simulink model "testHierCtrl"  (R2020a)
settings: Solver=FixedStepAuto  StartTime=0.0  StopTime=inf  FixedStep=0.01  RelTol=1e-3  EnableMultiTasking=on
values from neighbouring files (symbols this model uses):
  FLIGHTCONTROLLER = 'periodicCtrlExp'    [openWaterInit.m]
undefined symbols (not defined in the file or in its folder): env, fltCtrl, hiLvlCtrl, initializeBussesFromBlock, vhcl
libraries: simulink x6, filteredPIDController_ul x2, velocityAngle_ul x2, eeGeneralControl x1, stopwatch_ul x1, courseFollowManta_cl x1, ctrlAllocMatrix_cl x1, eulAng2RotMat_ul x1, angleBtw2Vecs_ul x1, vrlib x1, alphaBeta_ul x1, gnd2TanRotation_ul x1
settings Model: SimulationMode=external  Creator=andre  LastModifiedBy=mae-vermillionlab
settings SolverCC: ConcurrentTasks=on  AutoInsertRateTranBlk=on
settings DataIOCC: SaveFormat=StructureWithTime
settings OptimizationCC: BlockReduction=off  OptimizeBlockIOStorage=off
settings HardwareCC: ProdBitPerPointer=32  ProdBitPerSizeT=32  ProdBitPerPtrDiffT=32  ProdLargestAtomicFloat=None  ProdWordSize=32  ProdLongLongMode=on  ProdHWDeviceType=Generic->32-bit x86 compatible
settings RTWCC: Description=Simulink Real-Time  SystemTargetFile=slrt.tlc  TemplateMakefile=slrt_default_tmf  CodeExecutionProfiling=on  RTWCompilerOptimization=on
settings SimulinkRealTimeCC: SupportVariableSizeSignals=on  RL32LogTETModifier=off  xPCConcurrentTasks=on

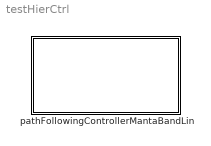
== system testHierCtrl ==
  pathFollowingControllerMantaBandLin : Subsystem  LoadFcn=initializeBussesFromBlock(gcb)  InitFcn=initializeBussesFromBlock(gcb)  StartFcn=initializeBussesFromBlock(gcb)  VariantControl=strcmpi(FLIGHTCONTROLLER,'pathFollowingControllerMantaBandLin')  mask{initPosForInitSStar=vhcl.initPosVecGnd.Value, fluidDensity=env.water.density.Value, pathCtrl=fltCtrl, aeroStruct=vhcl.struct('OCT.aeroSurf')}
      mask prompts: initPosForInitSStar "Initial Position"; fluidDensity "Fluid Density"; pathCtrl "Controller"; aeroStruct "Aerodynamic Structure"
      settings: MinAlgLoopOccurrences=on
      mask DialogControl Container3 Prompt: courseFollow Params
      mask DialogControl Container4 Prompt: setpointToOutput Params

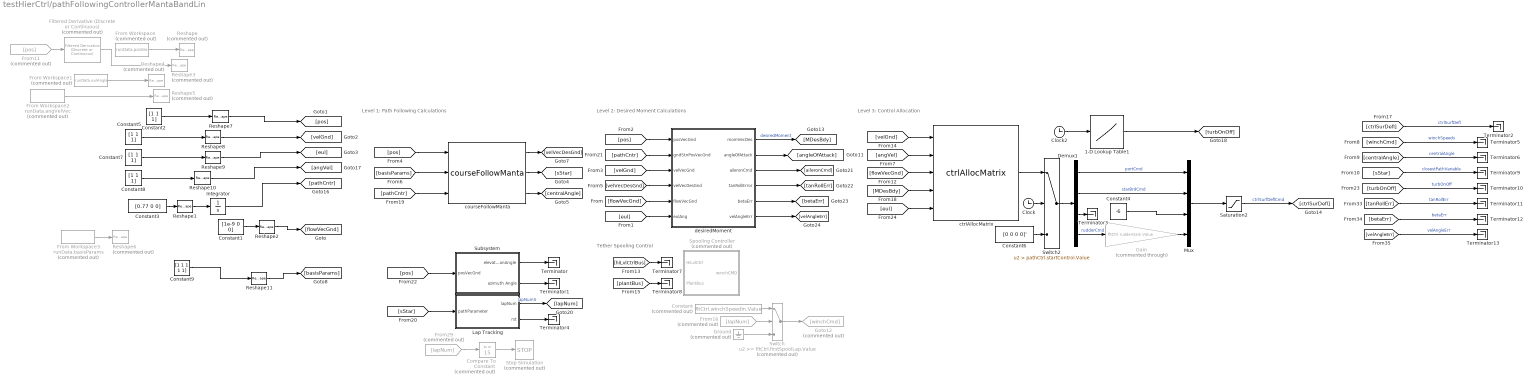
== system testHierCtrl/pathFollowingControllerMantaBandLin ==
  note: Level 1: Path Following Calculations
  note: Level 2: Desired Moment Calculations
  note: Tether Spooling Control
  note: Level 3: Control Allocation
  1-D Lookup Table1 : Lookup_n-D  NumberOfTableDimensions=1  BreakpointsForDimension1=[0 1000 2000]  Table=[0 0 0]  InterpMethod=Flat  InternalRulePriority=Speed  RndMeth=Simplest  InputSameDT=on
  Clock : Clock
  Clock2 : Clock
  Compare To Constant : simulink/Logic and Bit Operations/Compare To Constant  Commented=on  relop=>=  const=15  OutDataTypeStr=boolean
  Constant : Constant  Commented=on  Value=fltCtrl.winchSpeedIn.Value
  Constant1 : Constant  Value=[1e-9 0 0]
  Constant{2,5,7..8} (4 alike) : Constant  Value=[1 1 1]
  Constant3 : Constant  Value=[0.77 0 0]
  Constant4 : Constant  Value=-6
  Constant6 : Constant  Value=[0 0 0 0]'
  Constant9 : Constant  Value=[1 1 1 1 1]
  Demux1 : Demux
  Filtered Derivative (Discrete or Continuous) : eeGeneralControl/Filtered Derivative (Discrete or Continuous)  Commented=on  K=1  T=0.1  B=inf  A=-inf  minRatio=10  init_option=Inherited from block input  x0=0  Ts=-1
      settings: SourceProductBaseCode=PS
  From Workspace : FromWorkspace  Commented=on  VariableName=runData.posVec
  From Workspace1 : FromWorkspace  Commented=on  VariableName=runData.eulAngle
  From Workspace2 : FromWorkspace  Commented=on  VariableName=runData.angVelVec
  From Workspace3 : FromWorkspace  Commented=on  VariableName=runData.basisParams
  From11 : From  Commented=on  GotoTag=pos
  From16 : From  Commented=on  GotoTag=lapNum
  From29 : From  Commented=on  GotoTag=lapNum
  Gain : Gain  Commented=through  Gain=fltCtrl.rudderGain.Value
  Goto12 : Goto  Commented=on  GotoTag=winchCmd
  Ground : Ground  Commented=on
  Integrator : Integrator  InitialCondition=[0 0 0]'
  Lap Tracking : Subsystem
  Mux : Mux
  Reshape{,3..6} (5 alike) : Reshape  Commented=on  OutputDimensionality=Column vector (2-D)
  Reshape{1..2,7..11} (7 alike) : Reshape  OutputDimensionality=Column vector (2-D)
  Saturation2 : Saturate  UpperLimit=pathCtrl.controlSigMax.upperLimit.Value  LowerLimit=pathCtrl.controlSigMax.lowerLimit.Value
  "Spooling Controller " : Subsystem  Commented=on
  Stop Simulation : Stop  Commented=on
  Subsystem : Subsystem
  Switch : Switch  Commented=on  Threshold=fltCtrl.firstSpoolLap.Value
  Switch2 : Switch  Criteria=u2 > Threshold  Threshold=pathCtrl.startControl.Value
  Terminator{,1..13} (14 alike) : Terminator
  courseFollowManta : courseFollowManta_cl/courseFollowManta  SystemSampleTime=-1  Latency=0  AutoFrameSizeCalculation=off
      link override Memory1: InitialCondition=0
  ctrlAllocMatrix : ctrlAllocMatrix_cl/ctrlAllocMatrix  aeroStruct=aeroStruct  fluidDensity=fluidDensity
  desiredMoment : Subsystem
  wires:
  [velAngleErr] -> Terminator13/1  "velAngleErr"
  desiredMoment/6(velAngleErr) -> [velAngleErr]
  [betaErr] -> Terminator12/1  "betaErr"
  [tanRollErr] -> Terminator11/1  "tanRollErr"
  desiredMoment/5(betaErr) -> [betaErr]
  desiredMoment/4(tanRollError) -> [tanRollErr]
  Mux/1 -> Saturation2/1
  desiredMoment/3(aileronCmd) -> [aileronCmd]
  Compare To Constant/1 -> Stop Simulation/1
  From29/1 -> Compare To Constant/1
  Ground/1 -> Switch/3
  Constant/1 -> Switch/1
  From16/1 -> Switch/2
  Switch/1 -> Goto12/1
  [plantBus] -> Terminator8/1
  [hiLvlCtrlBus] -> Terminator7/1
  Lap Tracking/1(lapNum) -> [lapNum]  "lapNumS"
  Lap Tracking/2(rst) -> Terminator4/1
  [sStar] -> Lap Tracking/1(pathParameter)
  Clock2/1 -> 1-D Lookup Table1/1
  1-D Lookup Table1/1 -> [turbOnOff]
  desiredMoment/2(angleOfAttack) -> [angleOfAttack]
  Constant4/1 -> Mux/3
  Subsystem/2(azimuth Angle) -> Terminator1/1
  Subsystem/1(elevationAngle) -> Terminator/1
  [pos] -> Subsystem/1(posVecGnd)
  [turbOnOff] -> Terminator10/1  "turbOnOff"
  Demux1/4 -> Gain/1  "rudderCmd"
  Gain/1 -> Mux/4
  [basisParams] -> courseFollowManta/2
  [flowVecGnd] -> desiredMoment/5(flowVecGnd)
  [eul] -> desiredMoment/6(eulAng)
  [velVecDesGnd] -> desiredMoment/4(velVecDesGnd)
  [velGnd] -> desiredMoment/3(velVecGnd)
  [pathCntr] -> desiredMoment/2(gndStnPosVecGnd)
  [pos] -> desiredMoment/1(posVecGnd)
  [pathCntr] -> courseFollowManta/3
  [eul] -> ctrlAllocMatrix/5
  Saturation2/1 -> [ctrlSurDefl]  "ctrlSurfDeflCmd"
  [ctrlSurDefl] -> Terminator2/1  "ctrlSurfDefl"
  ctrlAllocMatrix/1 -> Switch2/1
  [MDesBdy] -> ctrlAllocMatrix/4
  Constant6/1 -> Switch2/3
  Switch2/1 -> Demux1/1
  Clock/1 -> Switch2/2
  Demux1/2 -> Mux/2  "starBrdCmd"
  Demux1/1 -> Mux/1  "portCmd"
  Demux1/3 -> Terminator3/1
  [flowVecGnd] -> ctrlAllocMatrix/3
  [velGnd] -> ctrlAllocMatrix/1
  [angVel] -> ctrlAllocMatrix/2
  desiredMoment/1(momVecDes) -> [MDesBdy]  "desiredMoment"
  courseFollowManta/3 -> [centralAngle]
  [sStar] -> Terminator9/1  "closestPathVariable"
  [centralAngle] -> Terminator6/1  "centralAngle"
  courseFollowManta/2 -> [sStar]
  [winchCmd] -> Terminator5/1  "winchSpeeds"
  [pos] -> courseFollowManta/1
  courseFollowManta/1 -> [velVecDesGnd]
  From Workspace/1 -> Reshape/1
  Filtered Derivative (Discrete or Continuous)/1 -> Reshape3/1
  From Workspace1/1 -> Reshape4/1
  Constant3/1 -> Reshape1/1
  Reshape1/1 -> Integrator/1
  Constant1/1 -> Reshape2/1
  Reshape2/1 -> [flowVecGnd]
  From11/1 -> Filtered Derivative (Discrete or Continuous)/1
  From Workspace2/1 -> Reshape5/1
  From Workspace3/1 -> Reshape6/1
  Reshape7/1 -> [pos]
  Constant2/1 -> Reshape7/1
  Constant5/1 -> Reshape8/1
  Constant7/1 -> Reshape9/1
  Constant8/1 -> Reshape10/1
  Integrator/1 -> [pathCntr]
  Reshape10/1 -> [angVel]
  Reshape9/1 -> [eul]
  Reshape8/1 -> [velGnd]
  Reshape11/1 -> [basisParams]
  Constant9/1 -> Reshape11/1

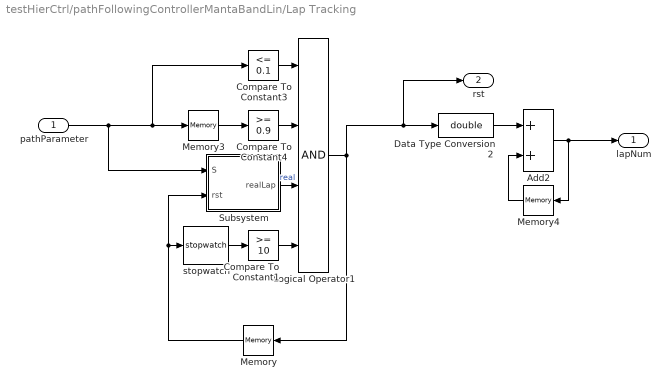
== system testHierCtrl/pathFollowingControllerMantaBandLin/Lap Tracking ==
  pathParameter : Inport
  Add2 : Sum
  Compare To Constant1 : simulink/Logic and Bit Operations/Compare To Constant  relop=>=  const=10  OutDataTypeStr=boolean
  Compare To Constant3 : simulink/Logic and Bit Operations/Compare To Constant  relop=<=  const=0.1  OutDataTypeStr=boolean
  Compare To Constant4 : simulink/Logic and Bit Operations/Compare To Constant  relop=>=  const=0.9  OutDataTypeStr=boolean
  Data Type Conversion2 : DataTypeConversion  OutDataTypeStr=double
  Logical Operator1 : Logic  Inputs=4  AllPortsSameDT=off  OutDataTypeStr=boolean
  Memory : Memory  InitialCondition=false
  Memory3 : Memory
  Memory4 : Memory
  Subsystem : Subsystem
  stopwatch : stopwatch_ul/stopwatch  SystemSampleTime=-1  Latency=0  AutoFrameSizeCalculation=off
  lapNum : Outport  VectorParamsAs1DForOutWhenUnconnected=off
  rst : Outport  Port=2  VectorParamsAs1DForOutWhenUnconnected=off
  wires:
  Subsystem/1(realLap) -> Logical Operator1/3  "real"
  Compare To Constant1/1 -> Logical Operator1/4
  Memory/1 -> stopwatch/1, Subsystem/2(rst)
  stopwatch/1 -> Compare To Constant1/1
  pathParameter/1 -> Memory3/1, Compare To Constant3/1, Subsystem/1(S)
  Compare To Constant4/1 -> Logical Operator1/2
  Add2/1 -> Memory4/1, lapNum/1
  Memory4/1 -> Add2/2
  Logical Operator1/1 -> Memory/1, Data Type Conversion2/1, rst/1
  Data Type Conversion2/1 -> Add2/1
  Memory3/1 -> Compare To Constant4/1
  Compare To Constant3/1 -> Logical Operator1/1

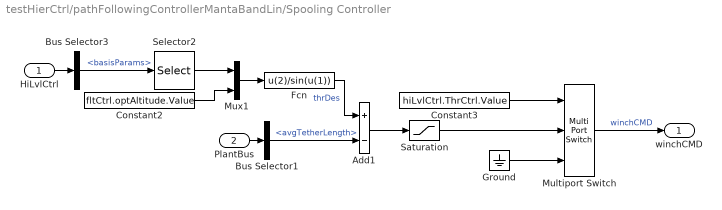
== system testHierCtrl/pathFollowingControllerMantaBandLin/Spooling Controller  ==
  HiLvlCtrl : Inport
  PlantBus : Inport  Port=2
  Add1 : Sum  Inputs=+-
  Bus Selector1 : BusSelector  OutputSignals=avgTetherLength
  Bus Selector3 : BusSelector  OutputSignals=basisParams
  Constant2 : Constant  Value=fltCtrl.optAltitude.Value
  Constant3 : Constant  Value=hiLvlCtrl.ThrCtrl.Value
  Fcn : Fcn  Expr=u(2)/sin(u(1))
  Ground : Ground
  Multiport Switch : MultiPortSwitch  DataPortOrder=Specify indices  Inputs=2  DataPortIndices={0,1}
  Mux1 : Mux  Inputs=2
  Saturation : Saturate  UpperLimit=.25  LowerLimit=-.25
  Selector2 : Selector  InputPortWidth=5  IndexOptions=Index vector (dialog)  Indices=3  OutputSizes=1
  winchCMD : Outport
  wires:
  PlantBus/1 -> Bus Selector1/1
  Constant3/1 -> Multiport Switch/1
  Saturation/1 -> Multiport Switch/2
  Ground/1 -> Multiport Switch/3
  HiLvlCtrl/1 -> Bus Selector3/1
  Multiport Switch/1 -> winchCMD/1  "winchCMD"
  Selector2/1 -> Mux1/1
  Fcn/1 -> Add1/1  "thrDes"
  Add1/1 -> Saturation/1
  Constant2/1 -> Mux1/2
  Bus Selector1/1 -> Add1/2  "<avgTetherLength>"
  Mux1/1 -> Fcn/1
  Bus Selector3/1 -> Selector2/1  "<basisParams>"

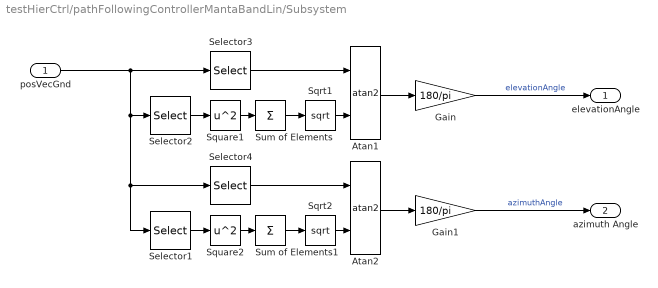
== system testHierCtrl/pathFollowingControllerMantaBandLin/Subsystem ==
  posVecGnd : Inport
  Atan1 : Trigonometry  Operator=atan2
  Atan2 : Trigonometry  Operator=atan2
  Gain : Gain  Gain=180/pi
  Gain1 : Gain  Gain=180/pi
  Selector1 : Selector  InputPortWidth=3  IndexOptions=Index vector (dialog)  Indices=1  OutputSizes=1
  Selector2 : Selector  InputPortWidth=3  IndexOptions=Index vector (dialog)  Indices=[1 2]  OutputSizes=1
  Selector3 : Selector  InputPortWidth=3  IndexOptions=Index vector (dialog)  Indices=3  OutputSizes=1
  Selector4 : Selector  InputPortWidth=3  IndexOptions=Index vector (dialog)  Indices=2  OutputSizes=1
  Sqrt1 : Sqrt  SaturateOnIntegerOverflow=on
  Sqrt2 : Sqrt  SaturateOnIntegerOverflow=on
  Square1 : Math  Operator=square  SignedPower=on  SaturateOnIntegerOverflow=on
  Square2 : Math  Operator=square  SignedPower=on  SaturateOnIntegerOverflow=on
  Sum of Elements : Sum  Inputs=+
  Sum of Elements1 : Sum  Inputs=+
  elevationAngle : Outport
  azimuth Angle : Outport  Port=2
  wires:
  Gain1/1 -> azimuth Angle/1  "azimuthAngle"
  Selector4/1 -> Atan2/1
  Sqrt2/1 -> Atan2/2
  posVecGnd/1 -> Selector3/1, Selector2/1, Selector4/1, Selector1/1
  Selector1/1 -> Square2/1
  Sum of Elements1/1 -> Sqrt2/1
  Square2/1 -> Sum of Elements1/1
  Atan2/1 -> Gain1/1
  Gain/1 -> elevationAngle/1  "elevationAngle"
  Selector2/1 -> Square1/1
  Atan1/1 -> Gain/1
  Sum of Elements/1 -> Sqrt1/1
  Selector3/1 -> Atan1/1
  Square1/1 -> Sum of Elements/1
  Sqrt1/1 -> Atan1/2

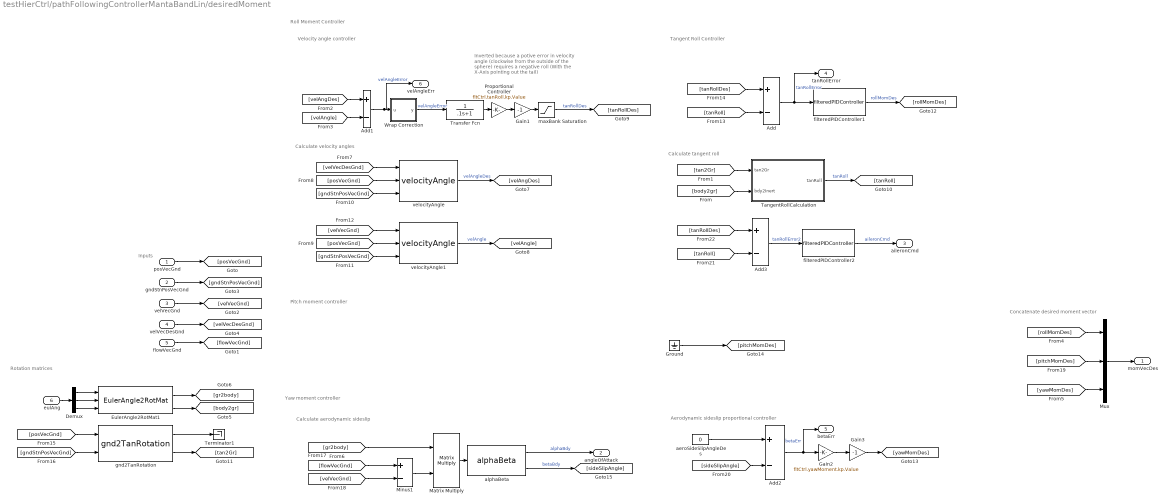
== system testHierCtrl/pathFollowingControllerMantaBandLin/desiredMoment ==
  note: Calculate aerodynamic sideslip
  note: Aerodynamic sideslip proportional controller
  note: Roll Moment Controller
  note: Concatenate desired moment vector
  note: Tangent Roll Controller
  note: Calculate tangent roll
  note: Calculate velocity angles
  note: Rotation matrices
  note: Inputs
  note: Velocity angle controller
  note: Inverted because a potive error
      | in velocity angle (clockwise from the
      | outside of the sphere) requires a negative
      | roll (With the X-Axis pointing out the tail)
  note: Pitch moment controller
  note: Yaw moment controller
  posVecGnd : Inport
  gndStnPosVecGnd : Inport  Port=2
  velVecGnd : Inport  Port=3
  velVecDesGnd : Inport  Port=4
  flowVecGnd : Inport  Port=5
  eulAng : Inport  Port=6
  Add{,1..3} (4 alike) : Sum  Inputs=+-
  Demux : Demux  Outputs=3
  EulerAngle2RotMat1 : eulAng2RotMat_ul/EulerAngle2RotMat  SystemSampleTime=-1  Latency=0  AutoFrameSizeCalculation=off
  Gain1 : Gain  Gain=-1
  Gain2 : Gain  Gain=fltCtrl.yawMoment.kp.Value
  Gain3 : Gain  Gain=-1
  Ground : Ground
  Matrix Multiply : Product  Multiplication=Matrix(*)
  Minus1 : Sum  Inputs=+-
  Mux : Mux  Inputs=3
  Proportional Controller : Gain  Gain=fltCtrl.tanRoll.kp.Value
  TangentRollCalculation : Subsystem
  Terminator1 : Terminator
  Transfer Fcn : TransferFcn  Denominator=[.1 1]
  Wrap Correction : Subsystem
  aeroSideSlipAngleDes : Constant  Value=0
  alphaBeta : alphaBeta_ul/alphaBeta  SystemSampleTime=-1  Latency=0  AutoFrameSizeCalculation=off
  filteredPIDController1 : filteredPIDController_ul/filteredPIDController  kp=pathCtrl.rollMoment.kp.Value  ki=0  kd=pathCtrl.rollMoment.kd.Value  Value=pathCtrl.rollMoment.tau.Value  externalReset=none
  filteredPIDController2 : filteredPIDController_ul/filteredPIDController  kp=fltCtrl.rollCtrl.kp.Value  ki=fltCtrl.rollCtrl.ki.Value  kd=fltCtrl.rollCtrl.kd.Value  Value=fltCtrl.rollCtrl.tau.Value  externalReset=none
  gnd2TanRotation : gnd2TanRotation_ul/gnd2TanRotation  SystemSampleTime=-1  Latency=0  AutoFrameSizeCalculation=off
  maxBank Saturation : Saturate  UpperLimit=pathCtrl.maxBank.upperLimit.Value  LowerLimit=pathCtrl.maxBank.lowerLimit.Value
  velocityAngle : velocityAngle_ul/velocityAngle  SystemSampleTime=-1  Latency=0  AutoFrameSizeCalculation=off
  velocityAngle1 : velocityAngle_ul/velocityAngle  SystemSampleTime=-1  Latency=0  AutoFrameSizeCalculation=off
  momVecDes : Outport  VectorParamsAs1DForOutWhenUnconnected=off
  angleOfAttack : Outport  Port=2  VectorParamsAs1DForOutWhenUnconnected=off
  aileronCmd : Outport  Port=3  VectorParamsAs1DForOutWhenUnconnected=off
  tanRollError : Outport  Port=4
  betaErr : Outport  Port=5
  velAngleErr : Outport  Port=6
  wires:
  filteredPIDController2/1 -> aileronCmd/1  "aileronCmd"
  [tanRollDes] -> Add3/1
  [tanRoll] -> Add3/2
  Add3/1 -> filteredPIDController2/1  "tanRollError2"
  Transfer Fcn/1 -> Proportional Controller/1
  Wrap Correction/1(y) -> Transfer Fcn/1  "velAngleError"
  Ground/1 -> [pitchMomDes]
  posVecGnd/1 -> [posVecGnd]
  velVecGnd/1 -> [velVecGnd]
  Add/1 -> filteredPIDController1/1, tanRollError/1  "tanRollError"
  Proportional Controller/1 -> Gain1/1
  Gain1/1 -> maxBank Saturation/1
  maxBank Saturation/1 -> [tanRollDes]  "tanRollDes"
  Add1/1 -> velAngleErr/1, Wrap Correction/1(u)  "velAngleError"
  flowVecGnd/1 -> [flowVecGnd]
  [tan2Gr] -> TangentRollCalculation/1(tan2Gr)
  TangentRollCalculation/1(tanRoll) -> [tanRoll]  "tanRoll"
  filteredPIDController1/1 -> [rollMomDes]  "rollMomDes"
  Gain2/1 -> Gain3/1
  Minus1/1 -> Matrix Multiply/2
  [velVecGnd] -> Minus1/2
  [flowVecGnd] -> Minus1/1
  eulAng/1 -> Demux/1
  Demux/3 -> EulerAngle2RotMat1/3
  Demux/1 -> EulerAngle2RotMat1/1
  Demux/2 -> EulerAngle2RotMat1/2
  EulerAngle2RotMat1/2 -> [body2gr]
  EulerAngle2RotMat1/1 -> [gr2body]
  [body2gr] -> TangentRollCalculation/2(bdy2Inert)
  [gr2body] -> Matrix Multiply/1
  Matrix Multiply/1 -> alphaBeta/1
  alphaBeta/2 -> [sideSlipAngle]  "betaBdy"
  Add2/1 -> Gain2/1, betaErr/1  "betaErr"
  aeroSideSlipAngleDes/1 -> Add2/1
  Mux/1 -> momVecDes/1
  Gain3/1 -> [yawMomDes]
  alphaBeta/1 -> angleOfAttack/1  "alphaBdy"
  [pitchMomDes] -> Mux/2
  gndStnPosVecGnd/1 -> [gndStnPosVecGnd]
  velVecDesGnd/1 -> [velVecDesGnd]
  velocityAngle/1 -> [velAngDes]  "velAngleDes"
  velocityAngle1/1 -> [velAngle]  "velAngle"
  [velAngDes] -> Add1/1
  [velAngle] -> Add1/2
  [velVecDesGnd] -> velocityAngle/1
  [posVecGnd] -> velocityAngle/2
  [posVecGnd] -> velocityAngle1/2
  [gndStnPosVecGnd] -> velocityAngle/3
  [gndStnPosVecGnd] -> velocityAngle1/3
  [velVecGnd] -> velocityAngle1/1
  [tanRoll] -> Add/2
  [tanRollDes] -> Add/1
  [posVecGnd] -> gnd2TanRotation/1
  [gndStnPosVecGnd] -> gnd2TanRotation/2
  gnd2TanRotation/2 -> [tan2Gr]
  gnd2TanRotation/1 -> Terminator1/1
  [rollMomDes] -> Mux/1
  [yawMomDes] -> Mux/3
  [sideSlipAngle] -> Add2/2

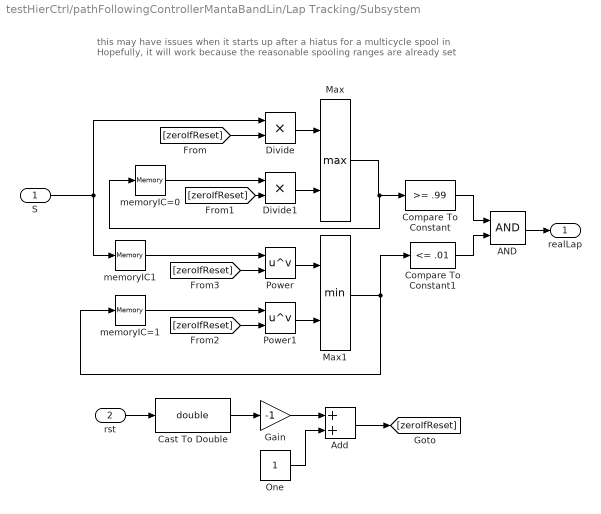
== system testHierCtrl/pathFollowingControllerMantaBandLin/Lap Tracking/Subsystem ==
  note: this may have issues when it starts up after a hiatus for a multicycle spool in
      | Hopefully, it will work because the reasonable spooling ranges are already set
  S : Inport
  rst : Inport  Port=2
  AND : Logic  AllPortsSameDT=off  OutDataTypeStr=boolean
  Add : Sum
  Cast To Double : DataTypeConversion  OutDataTypeStr=double
  Compare To Constant : simulink/Logic and Bit Operations/Compare To Constant  relop=>=  const=.99  OutDataTypeStr=boolean
  Compare To Constant1 : simulink/Logic and Bit Operations/Compare To Constant  relop=<=  const=.01  OutDataTypeStr=boolean
  Divide : Product  Inputs=**
  Divide1 : Product  Inputs=**
  Gain : Gain  Gain=-1
  Max : MinMax  Function=max  Inputs=2
  Max1 : MinMax  Inputs=2
  One : Constant  OutDataTypeStr=Inherit: Inherit via back propagation
  Power : Math  Operator=pow  SaturateOnIntegerOverflow=on
  Power1 : Math  Operator=pow  SaturateOnIntegerOverflow=on
  memoryIC1 : Memory  InitialCondition=1
  memoryIC=0 : Memory
  memoryIC=1 : Memory  InitialCondition=1
  realLap : Outport
  wires:
  memoryIC1/1 -> Power/1
  memoryIC=1/1 -> Power1/1
  [zeroIfReset] -> Power1/2
  memoryIC=0/1 -> Divide1/1
  Divide1/1 -> Max/2
  [zeroIfReset] -> Divide1/2
  [zeroIfReset] -> Power/2
  [zeroIfReset] -> Divide/2
  AND/1 -> realLap/1
  Compare To Constant1/1 -> AND/2
  Compare To Constant/1 -> AND/1
  Cast To Double/1 -> Gain/1
  Power1/1 -> Max1/2
  Power/1 -> Max1/1
  Max/1 -> Compare To Constant/1, memoryIC=0/1
  Divide/1 -> Max/1
  One/1 -> Add/2
  Add/1 -> [zeroIfReset]
  Gain/1 -> Add/1
  S/1 -> memoryIC1/1, Divide/1
  rst/1 -> Cast To Double/1
  Max1/1 -> memoryIC=1/1, Compare To Constant1/1

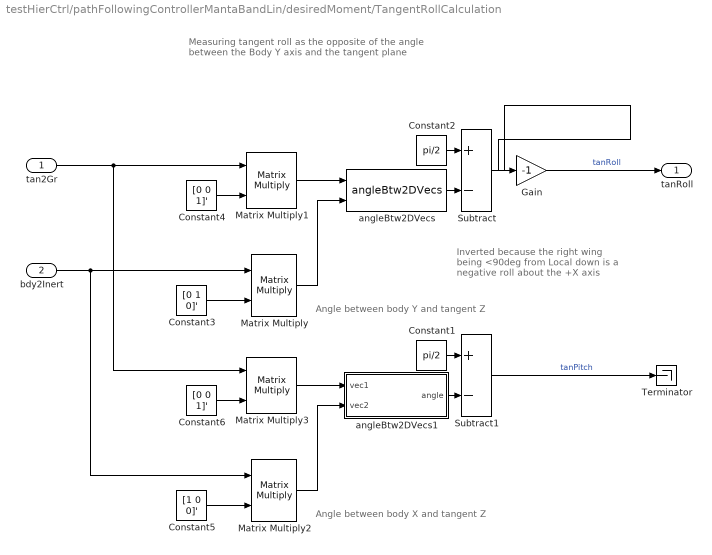
== system testHierCtrl/pathFollowingControllerMantaBandLin/desiredMoment/TangentRollCalculation ==
  note: Measuring tangent roll as the opposite
      | of the angle between the Body Y axis
      | and the tangent plane
  note: Angle between body Y and tangent Z
  note: Inverted because the right wing
      | being <90deg from Local down
      | is a negative roll about the +X axis
  note: Angle between body X and tangent Z
  tan2Gr : Inport
  bdy2Inert : Inport  Port=2
  Constant1 : Constant  Value=pi/2
  Constant2 : Constant  Value=pi/2
  Constant3 : Constant  Value=[0 1 0]'
  Constant4 : Constant  Value=[0 0 1]'
  Constant5 : Constant  Value=[1 0 0]'
  Constant6 : Constant  Value=[0 0 1]'
  Gain : Gain  Gain=-1
  Matrix Multiply{,1..3} (4 alike) : Product  Multiplication=Matrix(*)
  Subtract : Sum  Inputs=+-
  Subtract1 : Sum  Inputs=+-
  Terminator : Terminator
  angleBtw2DVecs : angleBtw2Vecs_ul/angleBtw2DVecs  SystemSampleTime=-1  Latency=0  AutoFrameSizeCalculation=off
  angleBtw2DVecs1 : Subsystem
  tanRoll : Outport  VectorParamsAs1DForOutWhenUnconnected=off
  wires:
  Subtract/1 -> Gain/1
  Constant3/1 -> Matrix Multiply/2
  angleBtw2DVecs/1 -> Subtract/2
  Constant2/1 -> Subtract/1
  Matrix Multiply1/1 -> angleBtw2DVecs/1
  Constant4/1 -> Matrix Multiply1/2
  Matrix Multiply/1 -> angleBtw2DVecs/2
  Gain/1 -> tanRoll/1  "tanRoll"
  bdy2Inert/1 -> Matrix Multiply2/1, Matrix Multiply/1
  Subtract1/1 -> Terminator/1  "tanPitch"
  tan2Gr/1 -> Matrix Multiply3/1, Matrix Multiply1/1
  Matrix Multiply2/1 -> angleBtw2DVecs1/2(vec2)
  Constant6/1 -> Matrix Multiply3/2
  Matrix Multiply3/1 -> angleBtw2DVecs1/1(vec1)
  Constant1/1 -> Subtract1/1
  angleBtw2DVecs1/1(angle) -> Subtract1/2
  Constant5/1 -> Matrix Multiply2/2

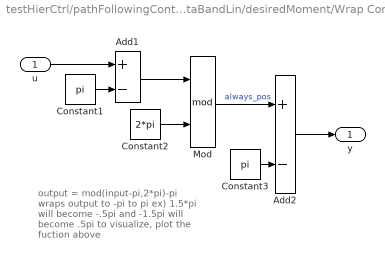
== system testHierCtrl/pathFollowingControllerMantaBandLin/desiredMoment/Wrap Correction ==
  note: output = mod(input-pi,2*pi)-pi
      | wraps output to -pi to pi
      |
      | ex) 1.5*pi will become -.5pi
      | 	and -1.5pi will become .5pi
      |
      | to visualize, plot the fuction above
  u : Inport
  Add1 : Sum  Inputs=+-
  Add2 : Sum  Inputs=+-
  Constant1 : Constant  Value=pi
  Constant2 : Constant  Value=2*pi
  Constant3 : Constant  Value=pi
  Mod : Math  Operator=mod  SignedPower=on  SaturateOnIntegerOverflow=on
  y : Outport  VectorParamsAs1DForOutWhenUnconnected=off
  wires:
  u/1 -> Add1/1
  Constant1/1 -> Add1/2
  Add1/1 -> Mod/1
  Constant2/1 -> Mod/2
  Mod/1 -> Add2/1  "always_pos"
  Constant3/1 -> Add2/2
  Add2/1 -> y/1

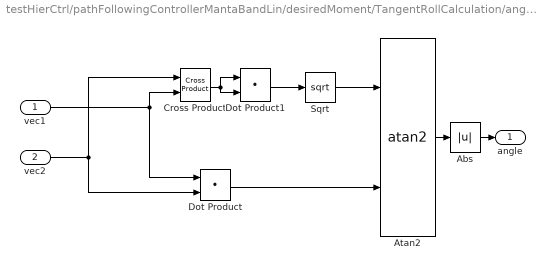
== system testHierCtrl/pathFollowingControllerMantaBandLin/desiredMoment/TangentRollCalculation/angleBtw2DVecs1 ==
  vec1 : Inport
  vec2 : Inport  Port=2
  Abs : Abs
  Atan2 : Trigonometry  Operator=atan2
  Cross Product : vrlib/Utilities/Cross Product
      settings: SourceProductBaseCode=VR
  Dot Product : DotProduct  InputSameDT=on  OutDataTypeStr=Inherit: Inherit via internal rule
  Dot Product1 : DotProduct  InputSameDT=on  OutDataTypeStr=Inherit: Inherit via internal rule
  Sqrt : Sqrt  SaturateOnIntegerOverflow=on
  angle : Outport  VectorParamsAs1DForOutWhenUnconnected=off
  wires:
  Atan2/1 -> Abs/1
  vec1/1 -> Dot Product/1, Cross Product/2
  vec2/1 -> Cross Product/1, Dot Product/2
  Cross Product/1 -> Dot Product1/1, Dot Product1/2
  Dot Product/1 -> Atan2/2
  Abs/1 -> angle/1
  Dot Product1/1 -> Sqrt/1
  Sqrt/1 -> Atan2/1
